simulink model "mmult"  (R2020a)
settings: Solver=VariableStepAuto  StartTime=0.0  StopTime=0  RelTol=1e-3  EnableMultiTasking=on
InitFcn:
  | setenv('DSPLIB_ROOT', './dsplib');
undefined symbols (not defined in the file): aie, blas, dsp, matrix_mult, matrix_mult_graph, xc7k325tffg900, xf
libraries: ModelComposer x3, simulink x1
settings Model: Creator=dvancamp  LastModifiedBy=abehbood
settings DataIOCC: ReturnWorkspaceOutputs=off
settings OptimizationCC: LifeSpan=inf
settings DebuggingCC: SFUnexpectedBacktrackingDiag=warning  SFNoUnconditionalDefaultTransitionDiag=warning  SFExecutionAtInitializationDiag=none  ArithmeticOperatorsInVariantConditions=warning
settings SFSimCC: SimUseLocalCustomCode=off  CustomCodeUndefinedFunction=UseInterfaceOnly
settings RTWCC: RTWUseLocalCustomCode=off
settings CodeAppCC: StateflowObjectComments=on
settings GRTTargetCC: TargetLangStandard=C89/C90 (ANSI)
settings ConfigComp: CovMetricSettings=dw  CovHtmlReporting=on  CovSaveCumulativeToWorkspaceVar=on  CovSaveSingleToWorkspaceVar=on  CovExternalEMLEnable=off

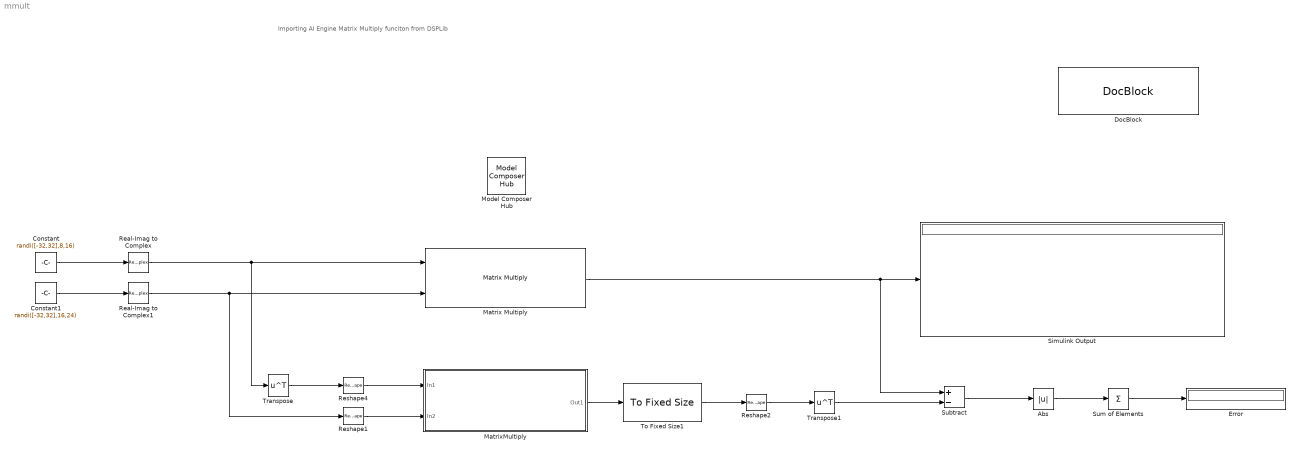
== system mmult ==
  note: Importing AI Engine Matrix Multiply funciton from DSPLib
  Abs : Abs
  Constant : Constant  Value=randi([-32,32],8,16)  OutDataTypeStr=int16  SampleTime=1
  Constant1 : Constant  Value=randi([-32,32],16,24)  OutDataTypeStr=int16  SampleTime=1
  DocBlock : simulink/Model-Wide Utilities/DocBlock  DocumentType=Text  mask(DocBlock){}
      content=|
      | ///////////////////////////////////////////////////////////////////////////
      | // Copyright 2021 Xilinx
      | //
      | // Licensed under the Apache License, Version 2.0 (the "License");
      | // you may not use this file except in compliance with the License.
      | // You may obtain a copy of the License at
      | //
      | // http://www.apache.org/licenses/LICENSE-2.0
      | //
      | // Unless required by applicable law or agreed to in writing, software
      | // distributed under the License is distributed on an "AS IS" BASIS,
      | // WITHOUT WARRANTIES OR CONDITIONS OF ANY KIND, either express or implied.
      | // See the License for the specific language governing permissions and
      | // limitations under the License.
      | ///////////////////////////////////////////////////////////////////////////
      mask Display:
      | xmcDrawBlockIcon();
      | disp(['{\fontsize{10pt}(c) Copyright 2021' ' Xilinx, Inc.}\newline \newline '],'texmode','on');
      | disp('{\fontsize{10pt}Licensed under the Apache License 2.0}','texmode','on');
      | disp('\newline \newline \newline{\fontsize{10pt}Double Click for Copyright Notice}','texmode','on');
  Error : Display
  Matrix Multiply : Product  Multiplication=Matrix(*)
  MatrixMultiply : Subsystem
      mask Display: xmcDrawAIEBlockIcon();
  Model Composer Hub : ModelComposer/Model Composer Hub  Description=Performs multiplication  CodeGeneration=off  SubsystemName=MatrixMultiply  TargetDirectory=./code  ExportType=AI Engines  IpVendor=xilinx.com  IpLibrary=hls  IpVersion=1.0  IpHWLanguage=Verilog  AieCompilerOptions={}  CreateTestbench=on  TestbenchStackSize=10  RunAieSim=on  AieSimTimeout=50000  RunAieSimProfiling=off  LaunchVitisAnalyzer=off  PlotOutput=off  RunX86Sim=on  X86SimTimeout=10  GenHwImage=off  PlatformType=Not Specified  ProjDevice=Kintex-7 KC705 Evaluation Platform (xc7k325tffg900-2)  ProjDevicePart=xc7k325tffg900-2  SamplePeriod=-1  ClockFrequency=200  DataPathParallelism=1
  Real-Imag to Complex : RealImagToComplex  Input=Real
  Real-Imag to Complex1 : RealImagToComplex  Input=Real
  Reshape1 : Reshape  OutputDimensions=[16,16]
  Reshape2 : Reshape  OutputDimensionality=Customize  OutputDimensions=[24,8]
  Reshape4 : Reshape  OutputDimensions=[16,16]
  Simulink Output : Display
  Subtract : Sum  Inputs=+-  OutDataTypeStr=double
  Sum of Elements : Sum  Inputs=+
  To Fixed Size1 : ModelComposer/To Fixed Size  OutputSize=192  CopyMethod=Pad with zeros or discard excess samples  HasStatusOutput=off
  Transpose : Math  Operator=transpose  SaturateOnIntegerOverflow=on
  Transpose1 : Math  Operator=transpose  SaturateOnIntegerOverflow=on
  wires:
  Constant1/1 -> Real-Imag to Complex1/1
  Constant/1 -> Real-Imag to Complex/1
  Transpose/1 -> Reshape4/1
  To Fixed Size1/1 -> Reshape2/1
  Reshape2/1 -> Transpose1/1
  Transpose1/1 -> Subtract/2
  Matrix Multiply/1 -> Subtract/1, Simulink Output/1
  Subtract/1 -> Abs/1
  Sum of Elements/1 -> Error/1
  Abs/1 -> Sum of Elements/1
  Real-Imag to Complex/1 -> Matrix Multiply/1, Transpose/1
  Real-Imag to Complex1/1 -> Matrix Multiply/2, Reshape1/1
  Reshape4/1 -> MatrixMultiply/1(In1)
  Reshape1/1 -> MatrixMultiply/2(In2)
  MatrixMultiply/1(Out1) -> To Fixed Size1/1

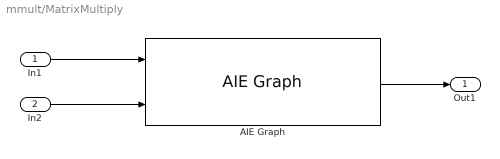
== system mmult/MatrixMultiply ==
  In1 : Inport
  In2 : Inport  Port=2
  AIE Graph : ModelComposer/AIE Graph  PortAttributesTable={'Input', 'inA[0]', 'window', 'cint16', '128', 'sync', '';'Input', 'inB[0]', 'window', 'cint16', '384', 'sync', '';'Output', 'out', 'window', 'cint16', '192', 'sync', ''}  PortAttributesEnablement={'off', 'on', 'off', 'off', 'off', 'off', 'off';'off', 'on', 'off', 'off', 'off', 'off', 'off';'off', 'on', 'off', 'off', 'off', 'off', 'off'}  SampleTime=-1  ClassDeclTypeOptions=C[2 1]@t354@template < typename TT_DATA_A, typename TT_DATA_B, int TP_DIM_A, int TP_DIM_AB, int TP_DIM_B, int TP_SHIFT, int TP_RND, int TP_DIM_A_LEADING, int TP_DIM_B_LEADING, int TP_DIM_OUT_LEADING, int TP_ADD_TILING_A, int TP_ADD_TILING_B, int TP_ADD_DETILING_OUT, int TP_INPUT_WINDOW_VSIZE_A, int TP_INPUT_WINDOW_VSIZE_B, int TP_CASC_LEN > class matrix_mult_grapht574@template < typename TT_DATA_A, typename TT_DATA_B, int TP_DIM_A, int TP_DIM_AB, int TP_DIM_B, int TP_SHIFT, int TP_RND, int TP_DIM_A_LEADING, int TP_DIM_B_LEADING, int TP_DIM_OUT_LEADING, int TP_ADD_TILING_A, int TP_ADD_TILING_B, int TP_ADD_DETILING_OUT, int TP_INPUT_WINDOW_VSIZE_A, int TP_INPUT_WINDOW_VSIZE_B > class matrix_mult_graph< TT_DATA_A, TT_DATA_B, TP_DIM_A, TP_DIM_AB, TP_DIM_B, TP_SHIFT, TP_RND, TP_DIM_A_LEADING, TP_DIM_B_LEADING, TP_DIM_OUT_LEADING, TP_ADD_TILING_A, TP_ADD_TILING_B, TP_ADD_DETILING_OUT, TP_INPUT_WINDOW_VSIZE_A, TP_INPUT_WINDOW_VSIZE_B, 1 >  ClassDecl=template < typename TT_DATA_A, typename TT_DATA_B, int TP_DIM_A, int TP_DIM_AB, int TP_DIM_B, int TP_SHIFT, int TP_RND, int TP_DIM_A_LEADING, int TP_DIM_B_LEADING, int TP_DIM_OUT_LEADING, int TP_ADD_TILING_A, int TP_ADD_TILING_B, int TP_ADD_DETILING_OUT, int TP_INPUT_WINDOW_VSIZE_A, int TP_INPUT_WINDOW_VSIZE_B, int TP_CASC_LEN > class matrix_mult_graph  ClassTemplateParams={'TT_DATA_A', 'typename', 'cint16';'TT_DATA_B', 'typename', 'cint16';'TP_DIM_A', 'int', '8';'TP_DIM_AB', 'int', '16';'TP_DIM_B', 'int', '24';'TP_SHIFT', 'int', '0';'TP_RND', 'int', '0';'TP_DIM_A_LEADING', 'int', 'ROW_MAJOR';'TP_DIM_B_LEADING', 'int', 'COL_MAJOR';'TP_DIM_OUT_LEADING', 'int', 'ROW_MAJOR';'TP_ADD_TILING_A', 'int', '1';'TP_ADD_TILING_B', 'int', '1';'TP_ADD_DETILING_OUT', 'int', '1';'TP_INPUT_WINDOW_VSIZE_A', 'int', '128';'TP_INPUT_WINDOW_VSIZE_B', 'int', '384';'TP_CASC_LEN', 'int', '1'}  ClassTemplateParamsEnables={'off', 'off', 'on';'off', 'off', 'on';'off', 'off', 'on';'off', 'off', 'on';'off', 'off', 'on';'off', 'off', 'on';'off', 'off', 'on';'off', 'off', 'on';'off', 'off', 'on';'off', 'off', 'on';'off', 'off', 'on';'off', 'off', 'on';'off', 'off', 'on';'off', 'off', 'on';'off', 'off', 'on';'off', 'off', 'on'}  ClassPortParams={ 'input', 'inA[TP_CASC_LEN]', 'off'; 'input', 'inB[TP_CASC_LEN]', 'off'; 'output', 'out', 'off' }  ClassCtorDeclTypeOptions=C[1 1]@t7@<empty>  ClassCtorDecl=<empty>  ClassCtorParams={}  GraphAllAttrs=|  PortArgDecls={'in window cint16 in1'; 'in window cint16 in2'; 'out window cint16 out1'}  PortGraphPortNames={'inA[0]'; 'inB[0]'; 'out'}  PortTypes={'window'; 'window'; 'window'}  PortDataTypes={'cint16'; 'cint16'; 'cint16'}  PortSizes={1.280000000000000000e+02; 3.840000000000000000e+02; 1.920000000000000000e+02}  PortSynchronicities={'sync'; 'sync'; 'sync'}  PortSignalSizes={0.000000000000000000e+00; 0.000000000000000000e+00; 0.000000000000000000e+00}  SimLibPath=''  ClassIndex=1  ClassCtorIndex=0  ClassTabVisible=on  FunctionTabVisible=on  GraphFileSelect=Header file (*.h)  GraphHeaderFile=dsplib/L2/include/hw/matrix_mult_graph.hpp  GraphClassName=xf::dsp::aie::blas::matrix_mult::matrix_mult_graph  GraphName=xf::dsp::aie::blas::matrix_mult::matrix_mult_graph<cint16, cint16, 8, 16, 24, 0, 0, 0, 1, 0, 1, 1, 1, 128, 384, 1>  GraphHeaderFiles={'dsplib/L2/include/hw/matrix_mult_graph.hpp'; 'dsplib/L2/include/hw/matrix_mult_tile_widget.hpp'}  GraphSourceFile=./model_composer_work/xmc_aie_lib/7c402d9b/mygraph.cpp  GraphSearchPaths={'$DSPLIB_ROOT/L1/include/hw', '$DSPLIB_ROOT/L2/include/hw', '$DSPLIB_ROOT/L1/src/hw', '$DSPLIB_ROOT/L1/tests/inc'}  GraphPreProcOptions={}  blockJsonConstraints=[]  deprecateConstraints=0
      | s[12;12;9;9;19;14;21;23;24;21;12;24;26;26;26;27;28;9;21;23;23;23;24;25;14;19;19;29]@FunctionNameDeclFileNamePortNamesPortTypesPortSerializedTypesPortDirectionsPortWindowSizeEnablesPortWindowMarginEnablesPortSynchronicityEnablesPortSignalSizeEnablesFunctionDeclFunctionTemplateSpecKindFunctionTemplateParamNamesFunctionTemplateParamKindsFunctionTemplateParamTypesFunctionTemplateParamValuesFunctionTemplateParamEnablesClassDeclClassTemplateSpecKindClassTemplateParamNamesClassTemplateParamKindsClassTemplateParamTypesClassTemplateParamValuesClassTemplateParamEnablesClassCtorDeclsClassCtorParamNamesClassCtorParamTypesClassCtorParamSerializedTypes[2 1]@C[28 2]@nt48@../../dsplib/L2/include/hw/matrix_mult_graph.hppC[3 1]@t3@inAt3@inBt3@outC[3 1]@t46@adf::port< adf::direction::in >[ TP_CASC_LEN ]t46@adf::port< adf::direction::in >[ TP_CASC_LEN ]t32@adf::port< adf::direction::out >C[3 1]@t53@{D{Tadf::port{1{t{Sadf::direction::in}}}}TP_CASC_LEN}t53@{D{Tadf::port{1{t{Sadf::direction::in}}}}TP_CASC_LEN}t40@{Tadf::port{1{t{Sadf::direction::out}}}}C[3 1]@t5@inputt5@inputt5@inputC[3 1]@l0@l0@l0@C[3 1]@l0@l0@l0@C[3 1]@l1@l1@l1@C[3 1]@l0@l0@l0@t600@namespace xf { namespace dsp { namespace aie { namespace blas { namespace matrix_mult {
      | template < typename TT_DATA_A, typename TT_DATA_B, int TP_DIM_A, int TP_DIM_AB, int TP_DIM_B, int TP_SHIFT, int TP_RND, int TP_DIM_A_LEADING, int TP_DIM_B_LEADING, int TP_DIM_OUT_LEADING, int TP_ADD_TILING_A, int TP_ADD_TILING_B, int TP_ADD_DETILING_OUT, int TP_INPUT_WINDOW_VSIZE_A, int TP_INPUT_WINDOW_VSIZE_B, int TP_CASC_LEN > 
      | void matrix_mult_graph::
      | (adf::port< adf::direction::in > inA [ TP_CASC_LEN ], adf::port< adf::direction::in > inB [ TP_CASC_LEN ], adf::port< adf::direction::out > out);
      | } } } } }ne[0 1]@e[0 1]@e[0 1]@e[0 1]@e[0 1]@t453@namespace xf { namespace dsp { namespace aie { namespace blas { namespace matrix_mult {
      | template < typename TT_DATA_A, typename TT_DATA_B, int TP_DIM_A, int TP_DIM_AB, int TP_DIM_B, int TP_SHIFT, int TP_RND, int TP_DIM_A_LEADING, int TP_DIM_B_LEADING, int TP_DIM_OUT_LEADING, int TP_ADD_TILING_A, int TP_ADD_TILING_B, int TP_ADD_DETILING_OUT, int TP_INPUT_WINDOW_VSIZE_A, int TP_INPUT_WINDOW_VSIZE_B, int TP_CASC_LEN > class matrix_mult_graph;
      | } } } } }t8@implicitC[16 1]@t9@TT_DATA_At9@TT_DATA_Bt8@TP_DIM_At9@TP_DIM_ABt8@TP_DIM_Bt8@TP_SHIFTt6@TP_RNDt16@TP_DIM_A_LEADINGt16@TP_DIM_B_LEADINGt18@TP_DIM_OUT_LEADINGt15@TP_ADD_TILING_At15@TP_ADD_TILING_Bt19@TP_ADD_DETILING_OUTt23@TP_INPUT_WINDOW_VSIZE_At23@TP_INPUT_WINDOW_VSIZE_Bt11@TP_CASC_LENC[16 1]@t4@typet4@typet7@nontypet7@nontypet7@nontypet7@nontypet7@nontypet7@nontypet7@nontypet7@nontypet7@nontypet7@nontypet7@nontypet7@nontypet7@nontypet7@nontypeC[16 1]@t8@typenamet8@typenamet3@intt3@intt3@intt3@intt3@intt3@intt3@intt3@intt3@intt3@intt3@intt3@intt3@intt3@intC[16 1]@nnnnnnnnnnnnnnnnC[16 1]@l1@l1@l1@l1@l1@l1@l1@l1@l1@l1@l1@l1@l1@l1@l1@l1@e[0 1]@e[0 1]@e[0 1]@e[0 1]@nt48@../../dsplib/L2/include/hw/matrix_mult_graph.hppC[3 1]@t3@inAt3@inBt3@outC[3 1]@t36@adf::port< adf::direction::in >[ 1 ]t36@adf::port< adf::direction::in >[ 1 ]t32@adf::port< adf::direction::out >C[3 1]@t43@{C{Tadf::port{1{t{Sadf::direction::in}}}}1}t43@{C{Tadf::port{1{t{Sadf::direction::in}}}}1}t40@{Tadf::port{1{t{Sadf::direction::out}}}}C[3 1]@t5@inputt5@inputt5@inputC[3 1]@l0@l0@l0@C[3 1]@l0@l0@l0@C[3 1]@l1@l1@l1@C[3 1]@l0@l0@l0@t800@namespace xf { namespace dsp { namespace aie { namespace blas { namespace matrix_mult {
      | template < typename TT_DATA_A, typename TT_DATA_B, int TP_DIM_A, int TP_DIM_AB, int TP_DIM_B, int TP_SHIFT, int TP_RND, int TP_DIM_A_LEADING, int TP_DIM_B_LEADING, int TP_DIM_OUT_LEADING, int TP_ADD_TILING_A, int TP_ADD_TILING_B, int TP_ADD_DETILING_OUT, int TP_INPUT_WINDOW_VSIZE_A, int TP_INPUT_WINDOW_VSIZE_B > 
      | void matrix_mult_graph< TT_DATA_A, TT_DATA_B, TP_DIM_A, TP_DIM_AB, TP_DIM_B, TP_SHIFT, TP_RND, TP_DIM_A_LEADING, TP_DIM_B_LEADING, TP_DIM_OUT_LEADING, TP_ADD_TILING_A, TP_ADD_TILING_B, TP_ADD_DETILING_OUT, TP_INPUT_WINDOW_VSIZE_A, TP_INPUT_WINDOW_VSIZE_B, 1 >::
      | (adf::port< adf::direction::in > inA [ 1 ], adf::port< adf::direction::in > inB [ 1 ], adf::port< adf::direction::out > out);
      | } } } } }ne[0 1]@e[0 1]@e[0 1]@e[0 1]@e[0 1]@t673@namespace xf { namespace dsp { namespace aie { namespace blas { namespace matrix_mult {
      | template < typename TT_DATA_A, typename TT_DATA_B, int TP_DIM_A, int TP_DIM_AB, int TP_DIM_B, int TP_SHIFT, int TP_RND, int TP_DIM_A_LEADING, int TP_DIM_B_LEADING, int TP_DIM_OUT_LEADING, int TP_ADD_TILING_A, int TP_ADD_TILING_B, int TP_ADD_DETILING_OUT, int TP_INPUT_WINDOW_VSIZE_A, int TP_INPUT_WINDOW_VSIZE_B > class matrix_mult_graph< TT_DATA_A, TT_DATA_B, TP_DIM_A, TP_DIM_AB, TP_DIM_B, TP_SHIFT, TP_RND, TP_DIM_A_LEADING, TP_DIM_B_LEADING, TP_DIM_OUT_LEADING, TP_ADD_TILING_A, TP_ADD_TILING_B, TP_ADD_DETILING_OUT, TP_INPUT_WINDOW_VSIZE_A, TP_INPUT_WINDOW_VSIZE_B, 1 >;
      | } } } } }t7@partialC[16 1]@t9@TT_DATA_At9@TT_DATA_Bt8@TP_DIM_At9@TP_DIM_ABt8@TP_DIM_Bt8@TP_SHIFTt6@TP_RNDt16@TP_DIM_A_LEADINGt16@TP_DIM_B_LEADINGt18@TP_DIM_OUT_LEADINGt15@TP_ADD_TILING_At15@TP_ADD_TILING_Bt19@TP_ADD_DETILING_OUTt23@TP_INPUT_WINDOW_VSIZE_At23@TP_INPUT_WINDOW_VSIZE_Bt11@TP_CASC_LENC[16 1]@t4@typet4@typet7@nontypet7@nontypet7@nontypet7@nontypet7@nontypet7@nontypet7@nontypet7@nontypet7@nontypet7@nontypet7@nontypet7@nontypet7@nontypet7@nontypeC[16 1]@t8@typenamet8@typenamet3@intt3@intt3@intt3@intt3@intt3@intt3@intt3@intt3@intt3@intt3@intt3@intt3@intt3@intC[16 1]@nnnnnnnnnnnnnnnt1@1C[16 1]@l1@l1@l1@l1@l1@l1@l1@l1@l1@l1@l1@l1@l1@l1@l1@l0@e[0 1]@e[0 1]@e[0 1]@e[0 1]@
  Out1 : Outport
  wires:
  In2/1 -> AIE Graph/2
  In1/1 -> AIE Graph/1
  AIE Graph/1 -> Out1/1
